simulink model "sscfluids_antagonistic_mckibben_actuator"  (R2019b)
settings: Solver=VariableStepAuto  StartTime=0.0  StopTime=10.0  RelTol=1e-3  AbsTol=1e-3  EnableMultiTasking=on
PreLoadFcn:
  | % Pressure source
  | p_source = 8e5; % Pa
  | 
  | % 4-way directional valve
  | valve_area_max = 3e-5; % m^2
  | L0 = 1e-5;
  | 
  | % Pipes
  | L_pipe = 20; % m
  | flow_area = 1e-4; % m^2
  | 
  | % Air muscle actuators
  | L_muscle = 30; % cm
  | L_braid = 32; % cm
  | n = 2.5;
  | 
  | % Flow control valves
  | dp_crack = 1e4; % Pa
  | dp_max = 2e4; % Pa
  | area_max = 1e-5; % m^2
  | area_leak = 1e-10; % m^2
  | area_restrict = 1e-6; % m^2
  | 
  | % Translational dampers
  | D_translation = 1; % N/(m/s)
  | 
  | % Translational hard stops
  | x_bound = 8; % cm
  | 
  | % Linkage
  | L_top = 15; % cm
  | L_bottom = 15; % cm
  | 
  | % Load
  | inertia = 0.005; % kg*m^2
  | D_rotation = 10; % N*m/(rad/s)
  | K_spring = 6.4; % N*m/rad
  | theta_upper = 0.4; % rad
  | theta_lower = 0; % rad
  | 
  | % Environment
  | T_atm = 293.15; % K
  | p_atm = 0.101325; % MPa
undefined symbols (not defined in the file): sigbuilder_block
libraries: fl_lib x24, SimscapeFluids_lib x7, fl_ps_legacy_lib x4, nesl_utility x4
(part 2 of 2)

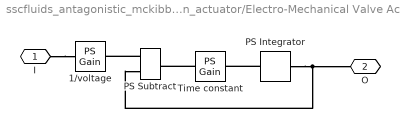
== system sscfluids_antagonistic_mckibben_actuator/Electro-Mechanical Valve Actuator ==
  1/voltage : fl_ps_legacy_lib/Legacy Physical Signals/Functions/PS Gain  gain=gain
      settings: SourceProductName=Simscape
  PS Integrator : fl_ps_legacy_lib/Legacy Physical Signals/Linear Operators/PS Integrator  x0=0
      settings: SourceProductName=Simscape  SourceProductBaseCode=SS  InternalSimscapePortConfiguration="{\"Bottom\":[],\"Left\":[{\"id\":\"I\",\"label\":\"\",\"type\":\"input\"}],\"Right\":[{\"id\":\"O\",\"label\":\"\",\"type\":\"output\"}],\"Top\":[]}"
  PS Subtract : fl_ps_legacy_lib/Legacy Physical Signals/Functions/PS Subtract
      settings: SourceProductName=Simscape  SourceProductBaseCode=SS
  Time constant : fl_ps_legacy_lib/Legacy Physical Signals/Functions/PS Gain  gain=1/time_const
      settings: SourceProductName=Simscape
  I : PMIOPort  Side=Left
  O : PMIOPort  Port=2  Side=Right
  connections:
  PS Integrator/RConn1 -- PS Subtract/LConn2 -- O/RConn1
  PS Subtract/LConn1 -- 1/voltage/RConn1
  I/RConn1 -- 1/voltage/LConn1
  PS Integrator/LConn1 -- Time constant/RConn1
  Time constant/LConn1 -- PS Subtract/RConn1

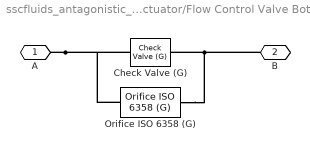
== system sscfluids_antagonistic_mckibben_actuator/Flow Control Valve Bottom ==
  Check Valve (G) : SimscapeFluids_lib/Gas/Valves & Orifices/Directional Control Valves/Check Valve (G)  pressure_spec=1  p_crack_differential=dp_crack Pa  p_crack_gauge=0.1 MPa  press_max_differential=dp_max Pa  press_max_gauge=0.2 MPa  iso_cond_spec=4  C_max=1.6 l/s/bar  C_min=1e-5 l/s/bar  B_crit=0.3  m=0.5  Cv_max=0.4  Cv_min=1e-6  Kv_max=0.3  Kv_min=1e-6  area_max=area_max m^2  area_leak=area_leak m^2  area=flow_area m^2  smoothing_factor=0.05  B_lam=0.999  T0=T_atm K  rho0=1.185 kg/m^3
      settings: SourceProductName=Simscape Fluids  SourceProductBaseCode=SH  InternalSimscapePortConfiguration="{\"Bottom\":[],\"Left\":[{\"id\":\"A\",\"label\":\"A\",\"type\":\"foundation.gas.gas\"}],\"Right\":[{\"id\":\"B\",\"label\":\"B\",\"type\":\"foundation.gas.gas\"}],\"Top\":[]}"
  Orifice ISO 6358 (G) : SimscapeFluids_lib/Gas/Valves & Orifices/Orifice ISO 6358 (G)  iso_cond_spec=4  C=1.6 l/s/bar  B_crit=0.3  m=0.5  Cv=0.4  Kv=0.3  restriction_area=area_restrict m^2  area=flow_area m^2  B_lam=0.999  T0=293.15 K  rho0=1.185 kg/m^3
      settings: SourceProductName=Simscape Fluids  SourceProductBaseCode=SH  InternalSimscapePortConfiguration="{\"Bottom\":[],\"Left\":[{\"id\":\"A\",\"label\":\"A\",\"type\":\"foundation.gas.gas\"}],\"Right\":[{\"id\":\"B\",\"label\":\"B\",\"type\":\"foundation.gas.gas\"}],\"Top\":[]}"
  A : PMIOPort  Side=Left
  B : PMIOPort  Port=2  Side=Right
  connections:
  A/RConn1 -- Orifice ISO 6358 (G)/LConn1 -- Check Valve (G)/LConn1
  B/RConn1 -- Orifice ISO 6358 (G)/RConn1 -- Check Valve (G)/RConn1

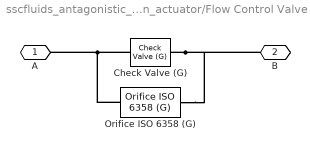
== system sscfluids_antagonistic_mckibben_actuator/Flow Control Valve Top ==
  Check Valve (G) : SimscapeFluids_lib/Gas/Valves & Orifices/Directional Control Valves/Check Valve (G)  pressure_spec=1  p_crack_differential=dp_crack Pa  p_crack_gauge=0.1 MPa  press_max_differential=dp_max Pa  press_max_gauge=0.2 MPa  iso_cond_spec=4  C_max=1.6 l/s/bar  C_min=1e-5 l/s/bar  B_crit=0.3  m=0.5  Cv_max=0.4  Cv_min=1e-6  Kv_max=0.3  Kv_min=1e-6  area_max=area_max m^2  area_leak=area_leak m^2  area=flow_area m^2  smoothing_factor=0.05  B_lam=0.999  T0=T_atm K  rho0=1.185 kg/m^3
      settings: SourceProductName=Simscape Fluids  SourceProductBaseCode=SH  InternalSimscapePortConfiguration="{\"Bottom\":[],\"Left\":[{\"id\":\"A\",\"label\":\"A\",\"type\":\"foundation.gas.gas\"}],\"Right\":[{\"id\":\"B\",\"label\":\"B\",\"type\":\"foundation.gas.gas\"}],\"Top\":[]}"
  Orifice ISO 6358 (G) : SimscapeFluids_lib/Gas/Valves & Orifices/Orifice ISO 6358 (G)  iso_cond_spec=4  C=1.6 l/s/bar  B_crit=0.3  m=0.5  Cv=0.4  Kv=0.3  restriction_area=area_restrict m^2  area=flow_area m^2  B_lam=0.999  T0=293.15 K  rho0=1.185 kg/m^3
      settings: SourceProductName=Simscape Fluids  SourceProductBaseCode=SH  InternalSimscapePortConfiguration="{\"Bottom\":[],\"Left\":[{\"id\":\"A\",\"label\":\"A\",\"type\":\"foundation.gas.gas\"}],\"Right\":[{\"id\":\"B\",\"label\":\"B\",\"type\":\"foundation.gas.gas\"}],\"Top\":[]}"
  A : PMIOPort  Side=Left
  B : PMIOPort  Port=2  Side=Right
  connections:
  Check Valve (G)/RConn1 -- Orifice ISO 6358 (G)/RConn1 -- B/RConn1
  Check Valve (G)/LConn1 -- Orifice ISO 6358 (G)/LConn1 -- A/RConn1

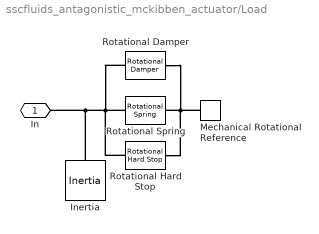
== system sscfluids_antagonistic_mckibben_actuator/Load ==
  Inertia : fl_lib/Mechanical/Rotational Elements/Inertia  inertia=inertia kg*m^2  w_specify=off  w_priority=High  w=0 rad/s  w_nominal_specify=off  w_nominal_unit=rad/s  w_nominal_value=1  t_specify=off  t_priority=None  t=0 N*m  t_nominal_specify=off  t_nominal_unit=N*m  t_nominal_value=1
  Mechanical Rotational Reference : fl_lib/Mechanical/Rotational Elements/Mechanical Rotational Reference
  Rotational Damper : fl_lib/Mechanical/Rotational Elements/Rotational Damper  D=D_rotation N*m/(rad/s)  w_specify=off  w_priority=None  w=0 rad/s  w_nominal_specify=off  w_nominal_unit=rad/s  w_nominal_value=1  t_specify=off  t_priority=None  t=0 N*m  t_nominal_specify=off  t_nominal_unit=N*m  t_nominal_value=1
  Rotational Hard Stop : fl_lib/Mechanical/Rotational Elements/Rotational Hard Stop  upper_bnd=theta_upper rad  lower_bnd=theta_lower rad  stiff_up=1e6 N*m/rad  stiff_low=1e6 N*m/rad  D_up=D_rotation N*m/(rad/s)  D_low=D_rotation N*m/(rad/s)  model=1  transition=0.001 rad  w_specify=off  w_priority=None  w=0 rad/s  w_nominal_specify=off  w_nominal_unit=rad/s  w_nominal_value=1  t_specify=off  t_priority=None  t=0 N*m  t_nominal_specify=off  t_nominal_unit=N*m  t_nominal_value=1  phi_specify=off  phi_priority=High  phi=0 rad  phi_nominal_specify=off  phi_nominal_unit=rad  phi_nominal_value=1
      settings: SourceProductName=Simscape  SourceProductBaseCode=SS
  Rotational Spring : fl_lib/Mechanical/Rotational Elements/Rotational Spring  spr_rate=K_spring N*m/rad  w_specify=off  w_priority=None  w=0 rad/s  w_nominal_specify=off  w_nominal_unit=rad/s  w_nominal_value=1  t_specify=off  t_priority=None  t=0 N*m  t_nominal_specify=off  t_nominal_unit=N*m  t_nominal_value=1  phi_specify=off  phi_priority=High  phi=0 rad  phi_nominal_specify=off  phi_nominal_unit=rad  phi_nominal_value=1
      settings: SourceProductName=Simscape
  In : PMIOPort  Side=Left
  connections:
  Rotational Spring/LConn1 -- Rotational Damper/LConn1 -- Rotational Hard Stop/LConn1 -- In/RConn1 -- Inertia/LConn1
  Mechanical Rotational Reference/LConn1 -- Rotational Hard Stop/RConn1 -- Rotational Damper/RConn1 -- Rotational Spring/RConn1

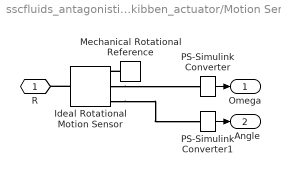
== system sscfluids_antagonistic_mckibben_actuator/Motion Sensor ==
  Ideal Rotational Motion Sensor : fl_lib/Mechanical/Mechanical Sensors/Ideal Rotational Motion Sensor  offset=0 rad
  Mechanical Rotational Reference : fl_lib/Mechanical/Rotational Elements/Mechanical Rotational Reference
  PS-Simulink Converter : nesl_utility/PS-Simulink Converter  PhysicalDomain=network_engine_domain  SubClassName=ps_output  LeftPortType=input  RightPortType=output  PseudoPeriodic=off  Frequencies=[]  Unit=1  AffineConversion=off
  PS-Simulink Converter1 : nesl_utility/PS-Simulink Converter  PhysicalDomain=network_engine_domain  SubClassName=ps_output  LeftPortType=input  RightPortType=output  PseudoPeriodic=off  Frequencies=[]  Unit=deg  AffineConversion=off
  R : PMIOPort  Side=Left
  Omega : Outport  VectorParamsAs1DForOutWhenUnconnected=off
  Angle : Outport  Port=2  VectorParamsAs1DForOutWhenUnconnected=off
  wires:
  PS-Simulink Converter1/1 -> Angle/1
  PS-Simulink Converter/1 -> Omega/1
  connections:
  Ideal Rotational Motion Sensor/RConn2 -- PS-Simulink Converter/LConn1
  Ideal Rotational Motion Sensor/RConn3 -- PS-Simulink Converter1/LConn1
  Mechanical Rotational Reference/LConn1 -- Ideal Rotational Motion Sensor/RConn1
  Ideal Rotational Motion Sensor/LConn1 -- R/RConn1

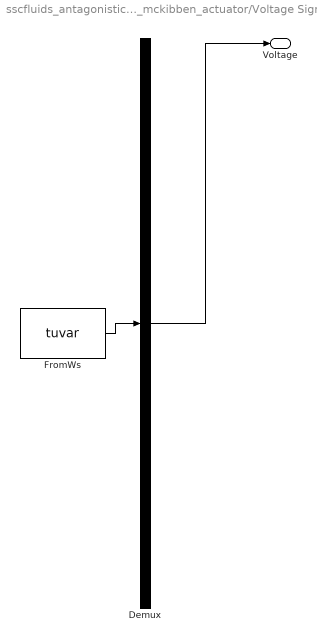
== system sscfluids_antagonistic_mckibben_actuator/Voltage Signal ==
  Demux : Demux  Tag=STV Demux  Outputs=1
  FromWs : FromWorkspace  Tag=STV FromWs  VariableName=tuvar  SampleTime=0
      SigBuilderData=|
      | common.afterFinalStr = 'Extrapolate'
      | common.sampleTime = 0
      | dataSet.timeRange = [0 10]
      | dataSet.name = 'V'
      | sbobj.Groups.Name = 'V'
      | sbobj.Groups.Signals.Name = 'Voltage'
      | sbobj.Groups.Signals.XData = [0 1 1.3 2.7 3 4 4.3 5.7 6 7 7.3 8.7 9 10]
      | sbobj.Groups.Signals.YData = [-22 -22 25 25 -22 -22 25 25 -22 -22 25 25 -22 -22]
  Voltage : Outport  Tag=STV Outport  VectorParamsAs1DForOutWhenUnconnected=off
  wires:
  FromWs/1 -> Demux/1
  Demux/1 -> Voltage/1
